simulink model "gm_uz_axi_mytestIP"  (R2022a)
settings: Solver=FixedStepDiscrete  StartTime=0.0  StopTime=50/100e6  RelTol=1e-3
settings Model: Creator=go98noz  LastModifiedBy=go98noz
settings SolverCC: AlgebraicLoopSolver=TrustRegion
settings DataIOCC: LimitDataPoints=on  SaveOutput=off  SaveTime=off
settings OptimizationCC: BlockReduction=off  ConditionallyExecuteInputs=off  DefaultParameterBehavior=Inlined  LifeSpan=inf
settings DebuggingCC: AlgebraicLoopMsg=error  InheritedTsInSrcMsg=none  SingleTaskRateTransMsg=error  UnconnectedInputMsg=warning  UnconnectedOutputMsg=warning  UnconnectedLineMsg=warning  AllowSymbolicDim=off  StrictBusMsg=ErrorOnBusTreatedAsVector  SFUnexpectedBacktrackingDiag=warning  SFNoUnconditionalDefaultTransitionDiag=warning  SFExecutionAtInitializationDiag=none  SFMachineParentedDataDiag=warning  ArithmeticOperatorsInVariantConditions=warning
settings HardwareCC: ProdBitPerPointer=32  ProdBitPerSizeT=32  ProdBitPerPtrDiffT=32  ProdLargestAtomicFloat=None  ProdIntDivRoundTo=Undefined  ProdEndianess=Unspecified  ProdWordSize=32  ProdHWDeviceType=ASIC/FPGA->ASIC/FPGA  ProdEqTarget=off
settings SFSimCC: SimUseLocalCustomCode=off  CustomCodeUndefinedFunction=UseInterfaceOnly
settings RTWCC: RTWUseLocalCustomCode=off
settings CodeAppCC: StateflowObjectComments=on
settings GRTTargetCC: TargetLangStandard=C89/C90 (ANSI)
settings ConfigComp: CovScope=ReferencedModels  CovMetricSettings=dw  CovSaveCumulativeToWorkspaceVar=on  CovSaveSingleToWorkspaceVar=on  CovExternalEMLEnable=off  CovSFcnEnable=off

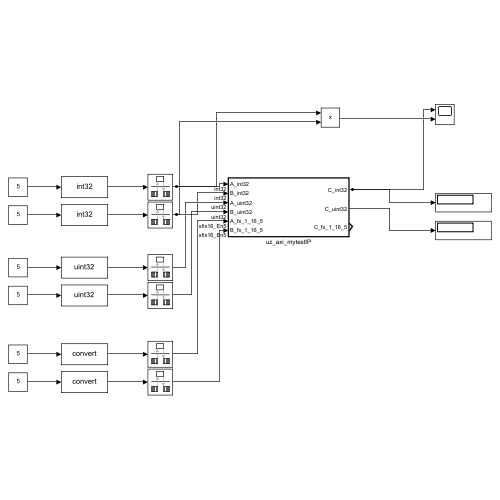
[thumbnail: Simulink's stored preview of the top-level diagram]
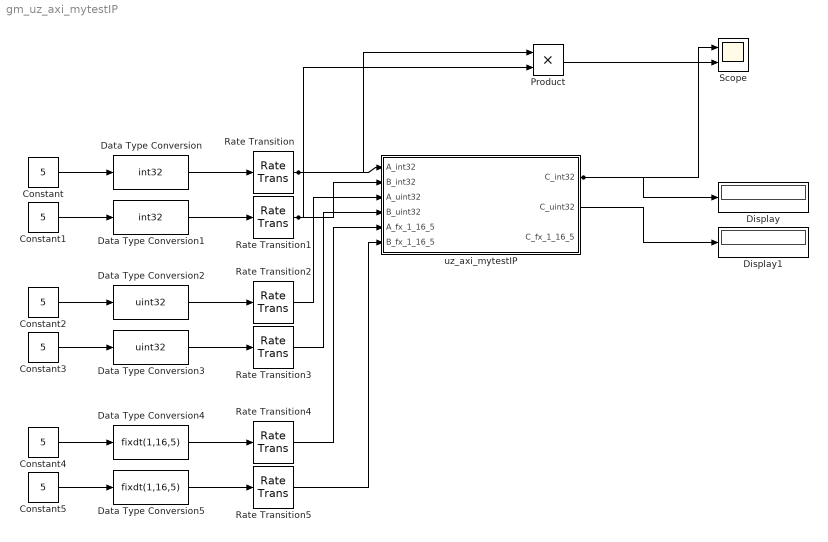
== system gm_uz_axi_mytestIP ==
  Constant{,1..5} (6 alike) : Constant  Value=5
  Data Type Conversion : DataTypeConversion  OutDataTypeStr=int32  SaturateOnIntegerOverflow=off  RndMeth=Floor
  Data Type Conversion1 : DataTypeConversion  OutDataTypeStr=int32  SaturateOnIntegerOverflow=off  RndMeth=Floor
  Data Type Conversion2 : DataTypeConversion  OutDataTypeStr=uint32  SaturateOnIntegerOverflow=off  RndMeth=Floor
  Data Type Conversion3 : DataTypeConversion  OutDataTypeStr=uint32  SaturateOnIntegerOverflow=off  RndMeth=Floor
  Data Type Conversion4 : DataTypeConversion  OutDataTypeStr=fixdt(1,16,5)  SaturateOnIntegerOverflow=off  RndMeth=Floor
  Data Type Conversion5 : DataTypeConversion  OutDataTypeStr=fixdt(1,16,5)  SaturateOnIntegerOverflow=off  RndMeth=Floor
  Display : Display
  Display1 : Display
  Product : Product  OutDataTypeStr=int32
  Rate Transition{,1..5} (6 alike) : RateTransition  OutPortSampleTime=1e-8
  Scope : Scope  NumInputPorts=2
  uz_axi_mytestIP : Subsystem  TreatAsAtomicUnit=on
  wires:
  Data Type Conversion5/1 -> Rate Transition5/1
  Data Type Conversion4/1 -> Rate Transition4/1
  Constant4/1 -> Data Type Conversion4/1
  Constant5/1 -> Data Type Conversion5/1
  Rate Transition4/1 -> uz_axi_mytestIP/5(A_fx_1_16_5)
  Rate Transition5/1 -> uz_axi_mytestIP/6(B_fx_1_16_5)
  uz_axi_mytestIP/2(C_uint32) -> Display1/1
  Rate Transition3/1 -> uz_axi_mytestIP/4(B_uint32)
  Rate Transition2/1 -> uz_axi_mytestIP/3(A_uint32)
  Constant3/1 -> Data Type Conversion3/1
  Constant2/1 -> Data Type Conversion2/1
  Data Type Conversion2/1 -> Rate Transition2/1
  Data Type Conversion3/1 -> Rate Transition3/1
  Product/1 -> Scope/2
  Rate Transition1/1 -> Product/2, uz_axi_mytestIP/2(B_int32)
  Rate Transition/1 -> uz_axi_mytestIP/1(A_int32), Product/1
  Data Type Conversion1/1 -> Rate Transition1/1
  Data Type Conversion/1 -> Rate Transition/1
  uz_axi_mytestIP/1(C_int32) -> Scope/1, Display/1
  Constant/1 -> Data Type Conversion/1
  Constant1/1 -> Data Type Conversion1/1

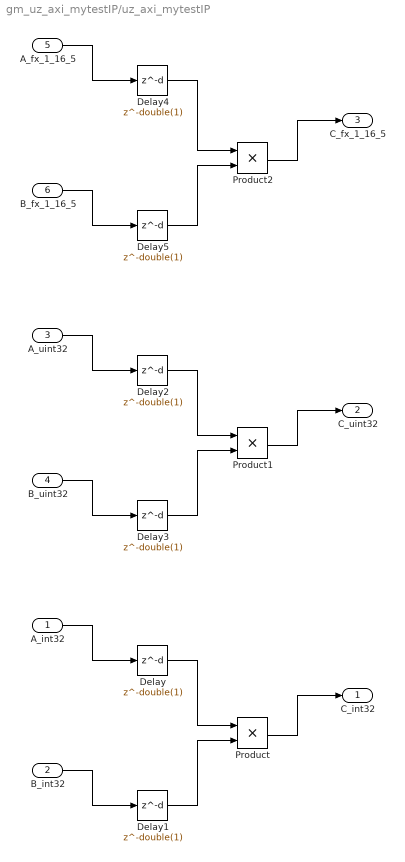
== system gm_uz_axi_mytestIP/uz_axi_mytestIP ==
  A_int32 : Inport  OutDataTypeStr=int32  PortDimensions=1  SampleTime=1e-08
  B_int32 : Inport  Port=2  OutDataTypeStr=int32  PortDimensions=1  SampleTime=1e-08
  A_uint32 : Inport  Port=3  OutDataTypeStr=uint32  PortDimensions=1  SampleTime=1e-08
  B_uint32 : Inport  Port=4  OutDataTypeStr=uint32  PortDimensions=1  SampleTime=1e-08
  A_fx_1_16_5 : Inport  Port=5  OutDataTypeStr=fixdt(1, 16, 5)  PortDimensions=1  SampleTime=1e-08
  B_fx_1_16_5 : Inport  Port=6  OutDataTypeStr=fixdt(1, 16, 5)  PortDimensions=1  SampleTime=1e-08
  Delay{,1..5} (6 alike) : Delay  DelayLength=double(1)  InitialCondition=0  SampleTime=1e-08
  Product : Product  Inputs=**  OutDataTypeStr=int32  SampleTime=1e-08
  Product1 : Product  Inputs=**  OutDataTypeStr=uint32  SampleTime=1e-08
  Product2 : Product  Inputs=**  OutDataTypeStr=fixdt(1, 16, 5)  SampleTime=1e-08
  C_int32 : Outport  SampleTime=1e-08  VectorParamsAs1DForOutWhenUnconnected=off
  C_uint32 : Outport  Port=2  SampleTime=1e-08  VectorParamsAs1DForOutWhenUnconnected=off
  C_fx_1_16_5 : Outport  Port=3  SampleTime=1e-08  VectorParamsAs1DForOutWhenUnconnected=off
  wires:
  A_int32/1 -> Delay/1
  B_int32/1 -> Delay1/1
  A_uint32/1 -> Delay2/1
  B_uint32/1 -> Delay3/1
  A_fx_1_16_5/1 -> Delay4/1
  B_fx_1_16_5/1 -> Delay5/1
  Delay/1 -> Product/1
  Delay1/1 -> Product/2
  Delay2/1 -> Product1/1
  Delay3/1 -> Product1/2
  Delay4/1 -> Product2/1
  Delay5/1 -> Product2/2
  Product/1 -> C_int32/1
  Product1/1 -> C_uint32/1
  Product2/1 -> C_fx_1_16_5/1
